simulink model "Modelo_COMPLETO_OPC"  (R2023a)
settings: Solver=ode15s  StartTime=0.0  StopTime=200  FixedStep=0.0001  MaxStep=0.01
model workspace (MAT data in the model file):
  socvcb = containers.Map
  socvcb.serialization.keys = {}
  socvcb.serialization.values = {}
  socvcb.serialization.uniformity = 0
  socvcb.serialization.keyType = 'double'
  socvcb.serialization.valueType = 'any'
undefined symbols (not defined in the file): b_cx, b_cy, b_hb, b_hd, b_hEb, b_hm, b_t, b_tb, b_td, b_tm, b_tw, b_wu, barco_x, barco_y, carro_y, constante_frenos, f, F_D_n_x, F_D_n_y, F_D_u_x, F_D_u_y, F_I_n_x, F_I_n_y, F_I_u_x, F_I_u_y, g, H_c, i_h, i_t, J_hdhEb, J_hmhb, J_td, J_tmtb, K_cy, K_tw, k_wu, M_s, M_t, muelle_x, muelle_y, pos_i_lh, pos_i_x, pos_i_yl, r_hd, r_td, riel_x, riel_y, T_hbMax, T_hEbMax, T_tbmax, xx_c0, Y_t0
libraries: simulink x6, opclib x3, vrlib x1
settings Model: Creator=Martin Tous  LastModifiedBy=Martin Tous
settings DebuggingCC: UnconnectedInputMsg=warning  UnconnectedOutputMsg=warning  UnconnectedLineMsg=warning
settings ModelReferenceCC: EnableRefExpFcnMdlSchedulingChecks=on
settings RTWCC: DLArmComputeVersion=19.05

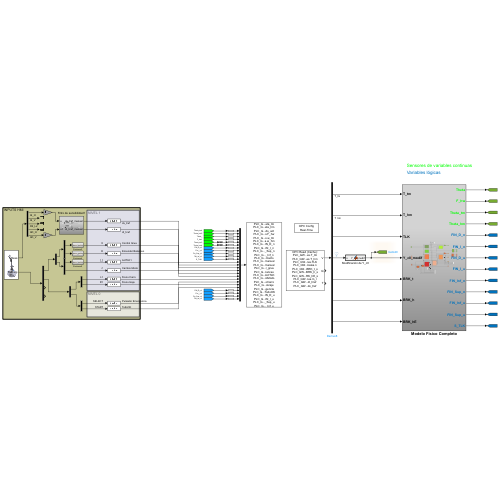
[thumbnail: Simulink's stored preview of the top-level diagram]
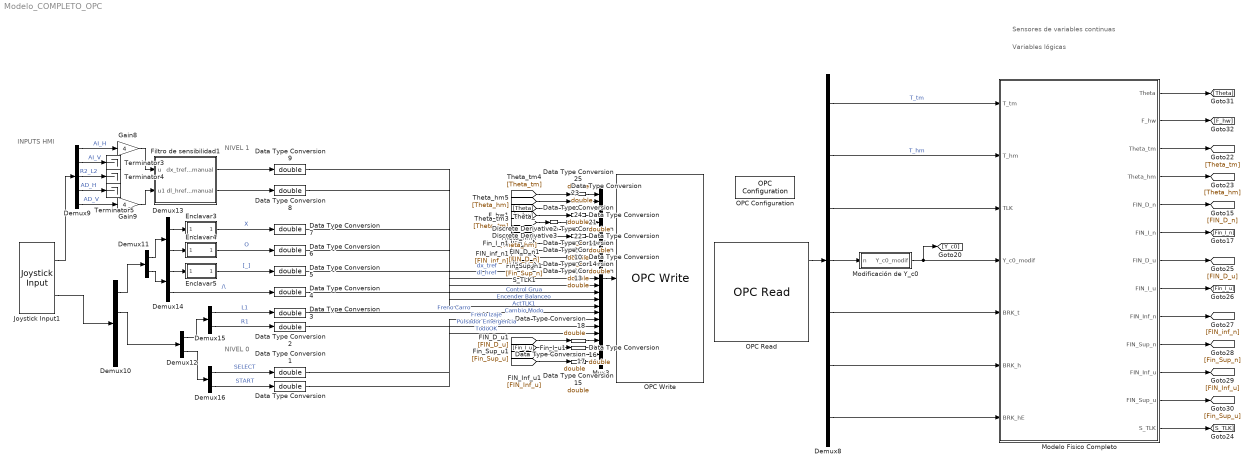
== system Modelo_COMPLETO_OPC ==
  note: INPUTS HMI
  note: NIVEL 0
  note: NIVEL 1
  note: Sensores de variables continuas
  note: Variables lógicas
  Data Type Conversion{,1..18,20..25} (25 alike) : DataTypeConversion  OutDataTypeStr=double  SaturateOnIntegerOverflow=off  RndMeth=Floor
  Demux10 : Demux
  Demux{11..16} (6 alike) : Demux  Outputs=2
  Demux8 : Demux  Outputs=7
  Demux9 : Demux  Outputs=5
  Discrete Derivative2 : simulink/Discrete/Discrete Derivative  gainval=1.0  ICPrevScaledInput=0.0  OutMin=[]  OutMax=[]  OutDataType=fixdt(1, 16)  OutScaling=2^-10  DoSatur=off
  Discrete Derivative3 : simulink/Discrete/Discrete Derivative  gainval=1.0  ICPrevScaledInput=0.0  OutMin=[]  OutMax=[]  OutDataType=fixdt(1, 16)  OutScaling=2^-10  DoSatur=off
  Enclavar3 : Stateflow chart  TreatAsAtomicUnit=on
  Enclavar4 : Stateflow chart  TreatAsAtomicUnit=on
  Enclavar5 : Stateflow chart  TreatAsAtomicUnit=on
  Filtro de sensibilidad1 : Subsystem
  Gain8 : Gain  Gain=4
  Gain9 : Gain  Gain=4
  Joystick Input1 : vrlib/Joystick Input  joyid=1  adjustports=on  forcefeed=off
  Modelo Fisico Completo : Subsystem
  Modificación de Y_c0 : MATLAB Function  TreatAsAtomicUnit=on
  Mux3 : Mux  Inputs=25
  OPC Configuration : opclib/OPC Configuration  opcServers=localhost/CoDeSys.OPC.DA/10  errMissingItems=Error  errReadWrite=Warn  errShutdown=Error  errRTViolation=Warn  rtEnable=on  speedup=1  showLatency=off  beingUsed=on
  OPC Read : opclib/OPC Read  serverHost=localhost  serverID=CoDeSys.OPC.DA  itemIDs=PLC_GW3.Application.Variables_Globales.T_tm, PLC_GW3.Application.Variables_Globales.T_hm, PLC_GW3.Application.Variables_Globales.TLK, PLC_GW3.Application.Variables_Globales.n, PLC_GW3.Application.Variables_Globales.BRK_t_s, PLC_GW3.Application.Variables_Globales.BRK_h_s, PLC_GW3.Application.Variables_Globales.BRK_hE_s, PLC_GW3.Application.Variables_Globales.m_l, PLC_GW3.Application.Variables_Globales.dl_href, PLC_GW3.Application.Variables_Globales.dx_tref  readMode=Synchronous (cache)  dataType=double  updateRate=0.01  showQual=on  showTS=on  tsMode=Seconds since start
  OPC Write : opclib/OPC Write  serverHost=localhost  serverID=CoDeSys.OPC.DA  itemIDs=PLC_GW3.Application.Variables_Globales.Theta_tm, PLC_GW3.Application.Variables_Globales.Theta_hm, PLC_GW3.Application.Variables_Globales.theta_realimentado_act, PLC_GW3.Application.Variables_Globales.F_hw, PLC_GW3.Application.Variables_Globales.w_tm, PLC_GW3.Application.Variables_Globales.w_hm, PLC_GW3.Application.Nivel1.FIN_D_n, PLC_GW3.Application.Nivel1.FIN_I_n, PLC_GW3.Application.Nivel1.FIN_Sup_n, PLC_GW3.Application.Nivel1.FIN_Inf_n, PLC_GW3.Application.Nivel1.SensoresContacto, PLC_GW3.Application.Nivel1.dx_tref_manual, PLC_GW3.Application.Nivel1.dl_href_manual, PLC_GW3.Application.Nivel1.Control_grua, PLC_GW3.Application.Nivel1.EncenderBalanceo, PLC_GW3.Application.Nivel1.ActTLK, PLC_GW3.Application.Nivel1.CambioModo, PLC_GW3.Application.Nivel1.BotonFrenoCarro, PLC_GW3.Application.Nivel1.BotonFrenoIzaje, PLC_GW3.Application.Nivel0.PulsadorEmergencia, PLC_GW3.Application.Nivel0.TodoOK, PLC_GW3.Application.Nivel0.FIN_D_u, PLC_GW3.Application.Nivel0.FIN_I_u, PLC_GW3.Application.Nivel0.FIN_Sup_u, PLC_GW3.Application.Nivel0.FIN_Inf_u  writeMode=Synchronous  updateRate=0.01
  Terminator3 : Terminator
  Terminator4 : Terminator
  Terminator5 : Terminator
  wires:
  Demux11/2 -> Demux14/1
  Demux16/1 -> Data Type Conversion1/1  "SELECT"
  Data Type Conversion3/1 -> Mux3/18  "Freno Carro"
  Data Type Conversion1/1 -> Mux3/20  "Pulsador Emergencia"
  Mux3/1 -> OPC Write/1
  Enclavar3/1(salida) -> Data Type Conversion7/1  "X"
  Filtro de sensibilidad1/1(dx_tref_manual) -> Data Type Conversion9/1
  Demux14/2 -> Data Type Conversion4/1  "/\\"
  Demux8/3 -> Modelo Fisico Completo/3(TLK)
  Demux10/1 -> Demux11/1
  Data Type Conversion6/1 -> Mux3/15  "Encender Balanceo"
  Demux14/1 -> Enclavar5/1(boton)
  Gain8/1 -> Filtro de sensibilidad1/1(u)
  Demux13/1 -> Enclavar3/1(boton)
  Demux9/3 -> Terminator4/1  "R2_L2"
  Demux9/5 -> Gain9/1  "AD_V"
  Demux13/2 -> Enclavar4/1(boton)
  Demux9/4 -> Terminator5/1  "AD_H"
  OPC Read/1 -> Demux8/1
  Gain9/1 -> Filtro de sensibilidad1/2(u1)
  Demux15/2 -> Data Type Conversion2/1  "R1"
  Demux11/1 -> Demux13/1
  Data Type Conversion7/1 -> Mux3/14  "Control Grua"
  Data Type Conversion5/1 -> Mux3/16  "ActTLK1"
  Filtro de sensibilidad1/2(dl_href_manual) -> Data Type Conversion8/1
  Demux10/2 -> Demux12/1
  Data Type Conversion2/1 -> Mux3/19  "Freno Izaje"
  Enclavar5/1(salida) -> Data Type Conversion5/1  "[_]"
  Demux12/1 -> Demux15/1
  Data Type Conversion/1 -> Mux3/21  "TodoOK"
  Demux12/2 -> Demux16/1
  Enclavar4/1(salida) -> Data Type Conversion6/1  "O"
  Demux9/2 -> Terminator3/1  "AI_V"
  Demux16/2 -> Data Type Conversion/1  "START"
  Data Type Conversion4/1 -> Mux3/17  "Cambio Modo"
  Demux9/1 -> Gain8/1  "AI_H"
  Joystick Input1/1 -> Demux9/1
  Demux15/1 -> Data Type Conversion3/1  "L1"
  Joystick Input1/2 -> Demux10/1
  [Fin_I_u] -> Data Type Conversion17/1
  [FIN_D_u] -> Data Type Conversion18/1
  [Fin_Sup_u] -> Data Type Conversion16/1
  [Fin_I_n] -> Data Type Conversion11/1
  [FIN_inf_n] -> Data Type Conversion13/1
  [Fin_Sup_n] -> Data Type Conversion12/1
  [S_TLK] -> Data Type Conversion14/1
  [FIN_D_n] -> Data Type Conversion10/1
  Data Type Conversion10/1 -> Mux3/7
  Data Type Conversion11/1 -> Mux3/8
  Data Type Conversion12/1 -> Mux3/9
  Data Type Conversion13/1 -> Mux3/10
  Data Type Conversion14/1 -> Mux3/11
  [FIN_Inf_u] -> Data Type Conversion15/1
  Data Type Conversion15/1 -> Mux3/25
  Data Type Conversion16/1 -> Mux3/24
  Data Type Conversion17/1 -> Mux3/23
  Data Type Conversion18/1 -> Mux3/22
  Discrete Derivative3/1 -> Data Type Conversion20/1
  [Theta_hm] -> Discrete Derivative3/1
  Discrete Derivative2/1 -> Data Type Conversion21/1
  [Theta_tm] -> Discrete Derivative2/1
  Data Type Conversion20/1 -> Mux3/6
  Data Type Conversion21/1 -> Mux3/5
  Data Type Conversion22/1 -> Mux3/4
  [F_hw] -> Data Type Conversion22/1
  Modelo Fisico Completo/8(FIN_I_u) -> [Fin_I_u]
  Modelo Fisico Completo/13(S_TLK) -> [S_TLK]
  Modelo Fisico Completo/5(FIN_D_n) -> [FIN_D_n]
  Modelo Fisico Completo/9(FIN_Inf_n) -> [FIN_inf_n]
  Modelo Fisico Completo/6(FIN_I_n) -> [Fin_I_n]
  Modelo Fisico Completo/2(F_hw) -> [F_hw]
  Modelo Fisico Completo/4(Theta_hm) -> [Theta_hm]
  Modelo Fisico Completo/10(FIN_Sup_n) -> [Fin_Sup_n]
  Modelo Fisico Completo/7(FIN_D_u) -> [FIN_D_u]
  Modelo Fisico Completo/1(Theta) -> [Theta]
  Modelo Fisico Completo/11(FIN_Inf_u) -> [FIN_Inf_u]
  Modelo Fisico Completo/12(FIN_Sup_u) -> [Fin_Sup_u]
  Modelo Fisico Completo/3(Theta_tm) -> [Theta_tm]
  Demux8/7 -> Modelo Fisico Completo/7(BRK_hE)
  Demux8/6 -> Modelo Fisico Completo/6(BRK_h)
  Demux8/5 -> Modelo Fisico Completo/5(BRK_t)
  Modificación de Y_c0/1(Y_c0_modif) -> Modelo Fisico Completo/4(Y_c0_modif), [Y_c0]
  [Theta] -> Data Type Conversion23/1
  Data Type Conversion23/1 -> Mux3/3
  Data Type Conversion25/1 -> Mux3/1
  Data Type Conversion24/1 -> Mux3/2
  [Theta_tm] -> Data Type Conversion25/1
  [Theta_hm] -> Data Type Conversion24/1
  Demux8/4 -> Modificación de Y_c0/1(n)
  Data Type Conversion8/1 -> Mux3/13  "dl_href"
  Data Type Conversion9/1 -> Mux3/12  "dx_tref"
  Demux8/1 -> Modelo Fisico Completo/1(T_tm)  "T_tm"
  Demux8/2 -> Modelo Fisico Completo/2(T_hm)  "T_hm"

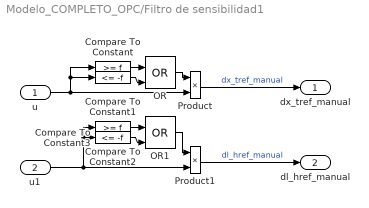
== system Modelo_COMPLETO_OPC/Filtro de sensibilidad1 ==
  u : Inport
  u1 : Inport  Port=2
  Compare To Constant : simulink/Logic and Bit Operations/Compare To Constant  relop=>=  const=f  OutDataTypeStr=boolean
  Compare To Constant1 : simulink/Logic and Bit Operations/Compare To Constant  relop=<=  const=-f  OutDataTypeStr=boolean
  Compare To Constant2 : simulink/Logic and Bit Operations/Compare To Constant  relop=>=  const=f  OutDataTypeStr=boolean
  Compare To Constant3 : simulink/Logic and Bit Operations/Compare To Constant  relop=<=  const=-f  OutDataTypeStr=boolean
  OR : Logic  Operator=OR  IconShape=distinctive  AllPortsSameDT=off  OutDataTypeStr=boolean
  OR1 : Logic  Operator=OR  IconShape=distinctive  AllPortsSameDT=off  OutDataTypeStr=boolean
  Product : Product
  Product1 : Product
  dx_tref_manual : Outport
  dl_href_manual : Outport  Port=2
  wires:
  u/1 -> Compare To Constant/1, Compare To Constant1/1, Product/2
  u1/1 -> Compare To Constant2/1, Compare To Constant3/1, Product1/2
  Compare To Constant1/1 -> OR/2
  Compare To Constant2/1 -> OR1/1
  Compare To Constant3/1 -> OR1/2
  OR1/1 -> Product1/1
  Compare To Constant/1 -> OR/1
  OR/1 -> Product/1
  Product/1 -> dx_tref_manual/1  "dx_tref_manual"
  Product1/1 -> dl_href_manual/1  "dl_href_manual"

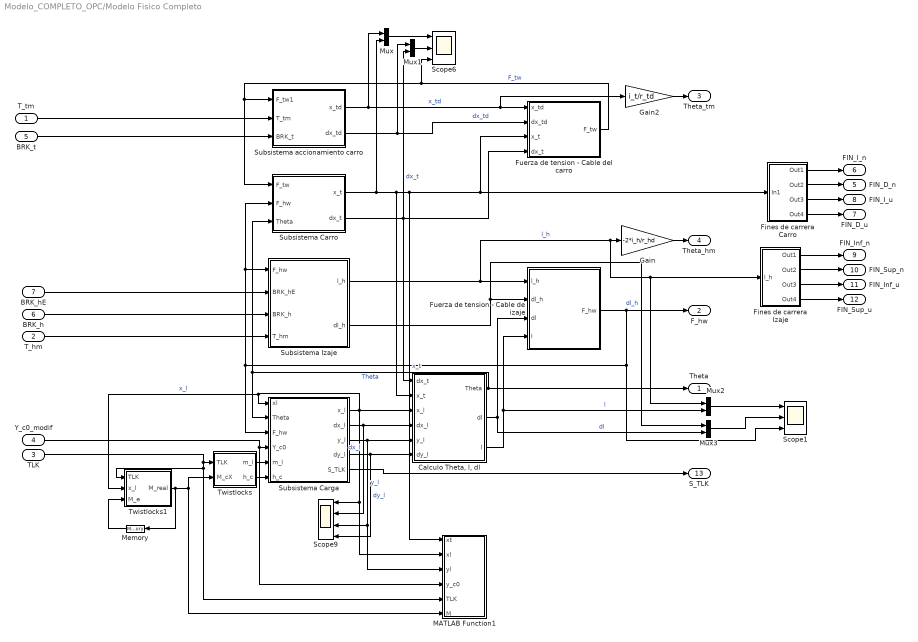
== system Modelo_COMPLETO_OPC/Modelo Fisico Completo ==
  T_tm : Inport
  T_hm : Inport  Port=2
  TLK : Inport  Port=3
  Y_c0_modif : Inport  Port=4
  BRK_t : Inport  Port=5
  BRK_h : Inport  Port=6
  BRK_hE : Inport  Port=7
  "Calculo Theta, l, dl" : Subsystem
  Fines de carrera Carro : Subsystem
  Fines de carrera Izaje : Subsystem
  Fuerza de tension - Cable de izaje : Subsystem
  Fuerza de tension - Cable del carro : Subsystem
  Gain : Gain  Gain=-2*i_h/r_hd
  Gain2 : Gain  Gain=i_t/r_td
  MATLAB Function1 : MATLAB Function  TreatAsAtomicUnit=on
  Memory : Memory
  Mux{,1..3} (4 alike) : Mux  Inputs=2
  Scope1 : Scope  NumInputPorts=3
  Scope6 : Scope  NumInputPorts=3
  Scope9 : Scope  NumInputPorts=4
  Subsistema Carga : Subsystem
  Subsistema Carro : Subsystem
  Subsistema Izaje : Subsystem
  Subsistema accionamiento carro : Subsystem
  Twistlocks : Stateflow chart  TreatAsAtomicUnit=on
  Twistlocks1 : Stateflow chart  TreatAsAtomicUnit=on
      settings: PortSchema="{\"entries\":[{\"content\":{\"sides\":[{\"content\":{\"connectorIds\":[\"In3\",\"In1\",\"In2\"]},\"type\":\"ConnectorPlacement.EquallySpacedRectSide\",\"uuid\":\"4fec8e6a-f8fa-4feb-a633-b12cd10cfa10\"},{\"content\":{\"connectorIds\":[\"Out1\"],\"side\":\"RIGHT\"},\"type\":\"ConnectorPlacement.EquallySpacedRectSide\",\"uuid\":\"3a43ccb0-d7f9-40a2-9c07-07991ad7e582\"},{\"content\":{\"connectorIds\":[],\"side\":\"TOP\"},\"type\":\"ConnectorPlacement.EquallySpacedRectSide\",\"uuid\":\"c629bb8f-87a5-4586-8b89-8bb15a2e67dc\"}]},\"type\":\"ConnectorPlacement.EquallySpacedConnector\",\"uuid\":\"e5885a79-67b0-4776-b045-dd8fc0c81e57\"}],\"packageUris\":[\"http://schema.mathworks.com/mf0/Connector/R2020b\"],\"version\":\"1.0\"}"
  Theta : Outport
  F_hw : Outport  Port=2
  Theta_tm : Outport  Port=3
  Theta_hm : Outport  Port=4
  FIN_D_n : Outport  Port=5
  FIN_I_n : Outport  Port=6
  FIN_D_u : Outport  Port=7
  FIN_I_u : Outport  Port=8
  FIN_Inf_n : Outport  Port=9
  FIN_Sup_n : Outport  Port=10
  FIN_Inf_u : Outport  Port=11
  FIN_Sup_u : Outport  Port=12
  S_TLK : Outport  Port=13
  wires:
  Fuerza de tension - Cable de izaje/1(F_hw) -> Subsistema Izaje/1(F_hw), Subsistema Carro/2(F_hw), Subsistema Carga/3(F_hw), Scope1/3, F_hw/1
  "Calculo Theta, l, dl"/1(Theta) -> Subsistema Carro/3(Theta), Subsistema Carga/2(Theta), Theta/1  "Theta"
  Subsistema Izaje/2(dl_h) -> Fuerza de tension - Cable de izaje/2(dl_h), Mux3/1  "dl_h"
  Twistlocks/1(m_l) -> Subsistema Carga/5(m_l)
  "Calculo Theta, l, dl"/2(dl) -> Mux3/2, Fuerza de tension - Cable de izaje/3(dl)  "dl"
  TLK/1 -> Twistlocks1/3(TLK), MATLAB Function1/5(TLK), Twistlocks/1(TLK)
  BRK_hE/1 -> Subsistema Izaje/2(BRK_hE)
  T_hm/1 -> Subsistema Izaje/4(T_hm)
  BRK_t/1 -> Subsistema accionamiento carro/3(BRK_t)
  BRK_h/1 -> Subsistema Izaje/3(BRK_h)
  Twistlocks/2(h_c) -> Subsistema Carga/6(h_c)
  T_tm/1 -> Subsistema accionamiento carro/2(T_tm)
  Gain2/1 -> Theta_tm/1
  Subsistema Izaje/1(l_h) -> Fuerza de tension - Cable de izaje/1(l_h), Mux2/1, Fines de carrera Izaje/1(l_h), Gain/1  "l_h"
  Gain/1 -> Theta_hm/1
  "Calculo Theta, l, dl"/3(l) -> Mux2/2, Fuerza de tension - Cable de izaje/4(l)  "l"
  Twistlocks1/1(M_real) -> Memory/1, Twistlocks/2(M_cX), MATLAB Function1/6(M)
  Subsistema Carro/2(dx_t) -> Mux1/2, Fuerza de tension - Cable del carro/4(dx_t), "Calculo Theta, l, dl"/1(dx_t)  "dx_t"
  Subsistema Carga/5(S_TLK) -> S_TLK/1
  Y_c0_modif/1 -> MATLAB Function1/4(y_c0), Subsistema Carga/4(Y_c0)
  Subsistema Carro/1(x_t) -> MATLAB Function1/1(xt), Fines de carrera Carro/1(In1), Fuerza de tension - Cable del carro/3(x_t), "Calculo Theta, l, dl"/2(x_t), Mux/2  "x_t"
  Fines de carrera Carro/1(Out1) -> FIN_I_n/1
  Fines de carrera Carro/2(Out2) -> FIN_D_n/1
  Fines de carrera Carro/3(Out3) -> FIN_I_u/1
  Fines de carrera Carro/4(Out4) -> FIN_D_u/1
  Fines de carrera Izaje/1(Out1) -> FIN_Inf_n/1
  Fines de carrera Izaje/2(Out2) -> FIN_Sup_n/1
  Fines de carrera Izaje/3(Out3) -> FIN_Inf_u/1
  Fines de carrera Izaje/4(Out4) -> FIN_Sup_u/1
  Fuerza de tension - Cable del carro/1(F_tw) -> Subsistema Carro/1(F_tw), Subsistema accionamiento carro/1(F_tw1), Scope6/3  "F_tw"
  Subsistema accionamiento carro/2(dx_td) -> Mux1/1, Fuerza de tension - Cable del carro/2(dx_td)  "dx_td"
  Subsistema accionamiento carro/1(x_td) -> Gain2/1, Fuerza de tension - Cable del carro/1(x_td), Mux/1  "x_td"
  Subsistema Carga/3(y_l) -> "Calculo Theta, l, dl"/5(y_l), Scope9/3, MATLAB Function1/3(yl)  "y_l"
  Subsistema Carga/2(dx_l) -> "Calculo Theta, l, dl"/4(dx_l), Scope9/2  "dx_l"
  Subsistema Carga/4(dy_l) -> "Calculo Theta, l, dl"/6(dy_l), Scope9/4  "dy_l"
  Subsistema Carga/1(x_l) -> "Calculo Theta, l, dl"/3(x_l), Scope9/1, MATLAB Function1/2(xl), Twistlocks1/1(x_l), Subsistema Carga/1(xl)  "x_l"
  Mux/1 -> Scope6/1
  Mux1/1 -> Scope6/2
  Mux2/1 -> Scope1/1
  Mux3/1 -> Scope1/2
  Memory/1 -> Twistlocks1/2(M_e)

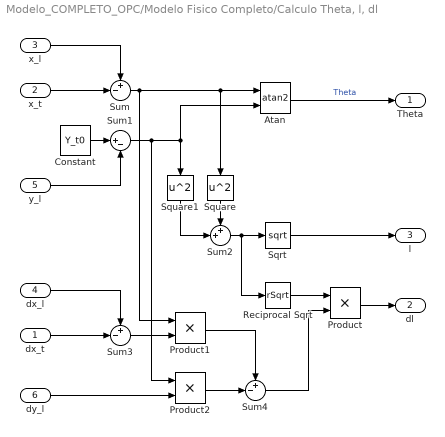
== system Modelo_COMPLETO_OPC/Modelo Fisico Completo/Calculo Theta, l, dl ==
  dx_t : Inport
  x_t : Inport  Port=2
  x_l : Inport  Port=3
  dx_l : Inport  Port=4
  y_l : Inport  Port=5
  dy_l : Inport  Port=6
  Atan : Trigonometry  Operator=atan2
  Constant : Constant  Value=Y_t0
  Product : Product
  Product1 : Product
  Product2 : Product
  Reciprocal Sqrt : Sqrt  Operator=rSqrt
  Sqrt : Sqrt
  Square : Math  Operator=square
  Square1 : Math  Operator=square
  Sum : Sum  Inputs=+-|
  Sum1 : Sum  Inputs=|+-
  Sum2 : Sum  Inputs=++|
  Sum3 : Sum  Inputs=+-|
  Sum4 : Sum  Inputs=+-|
  Theta : Outport
  dl : Outport  Port=2
  l : Outport  Port=3
  wires:
  y_l/1 -> Sum1/2
  Sum1/1 -> Product2/1, Square1/1, Atan/2
  Sum/1 -> Square/1, Atan/1, Product1/1
  Constant/1 -> Sum1/1
  Atan/1 -> Theta/1  "Theta"
  x_l/1 -> Sum/1
  x_t/1 -> Sum/2
  Square/1 -> Sum2/1
  Square1/1 -> Sum2/2
  Sum2/1 -> Reciprocal Sqrt/1, Sqrt/1
  Sqrt/1 -> l/1
  Reciprocal Sqrt/1 -> Product/1
  dx_l/1 -> Sum3/1
  dx_t/1 -> Sum3/2
  Sum3/1 -> Product1/2
  Product1/1 -> Sum4/1
  dy_l/1 -> Product2/2
  Product2/1 -> Sum4/2
  Sum4/1 -> Product/2
  Product/1 -> dl/1

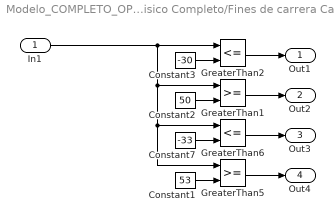
== system Modelo_COMPLETO_OPC/Modelo Fisico Completo/Fines de carrera Carro ==
  In1 : Inport
  Constant1 : Constant  Value=53
  Constant2 : Constant  Value=50
  Constant3 : Constant  Value=-30
  Constant7 : Constant  Value=-33
  GreaterThan1 : RelationalOperator  OutDataTypeStr=boolean  RndMeth=Simplest  InputSameDT=off
  GreaterThan2 : RelationalOperator  Operator=<=  OutDataTypeStr=boolean  RndMeth=Simplest  InputSameDT=off
  GreaterThan5 : RelationalOperator  OutDataTypeStr=boolean  RndMeth=Simplest  InputSameDT=off
  GreaterThan6 : RelationalOperator  Operator=<=  OutDataTypeStr=boolean  RndMeth=Simplest  InputSameDT=off
  Out1 : Outport
  Out2 : Outport  Port=2
  Out3 : Outport  Port=3
  Out4 : Outport  Port=4
  wires:
  GreaterThan1/1 -> Out2/1
  In1/1 -> GreaterThan5/1, GreaterThan6/1, GreaterThan1/1, GreaterThan2/1
  GreaterThan2/1 -> Out1/1
  Constant3/1 -> GreaterThan2/2
  Constant2/1 -> GreaterThan1/2
  Constant1/1 -> GreaterThan5/2
  Constant7/1 -> GreaterThan6/2
  GreaterThan6/1 -> Out3/1
  GreaterThan5/1 -> Out4/1

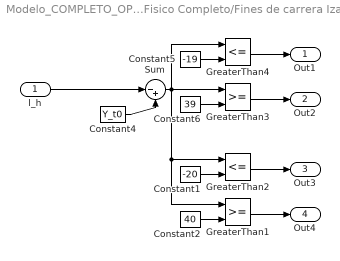
== system Modelo_COMPLETO_OPC/Modelo Fisico Completo/Fines de carrera Izaje ==
  l_h : Inport
  Constant1 : Constant  Value=-20
  Constant2 : Constant  Value=40
  Constant4 : Constant  Value=Y_t0
  Constant5 : Constant  Value=-19
  Constant6 : Constant  Value=39
  GreaterThan1 : RelationalOperator  OutDataTypeStr=boolean  RndMeth=Simplest  InputSameDT=off
  GreaterThan2 : RelationalOperator  Operator=<=  OutDataTypeStr=boolean  RndMeth=Simplest  InputSameDT=off
  GreaterThan3 : RelationalOperator  OutDataTypeStr=boolean  RndMeth=Simplest  InputSameDT=off
  GreaterThan4 : RelationalOperator  Operator=<=  OutDataTypeStr=boolean  RndMeth=Simplest  InputSameDT=off
  Sum : Sum  Inputs=|-+
  Out1 : Outport
  Out2 : Outport  Port=2
  Out3 : Outport  Port=3
  Out4 : Outport  Port=4
  wires:
  Constant1/1 -> GreaterThan2/2
  Sum/1 -> GreaterThan3/1, GreaterThan4/1, GreaterThan1/1, GreaterThan2/1
  Constant6/1 -> GreaterThan3/2
  Constant4/1 -> Sum/2
  Constant5/1 -> GreaterThan4/2
  Constant2/1 -> GreaterThan1/2
  GreaterThan3/1 -> Out2/1
  GreaterThan4/1 -> Out1/1
  l_h/1 -> Sum/1
  GreaterThan2/1 -> Out3/1
  GreaterThan1/1 -> Out4/1

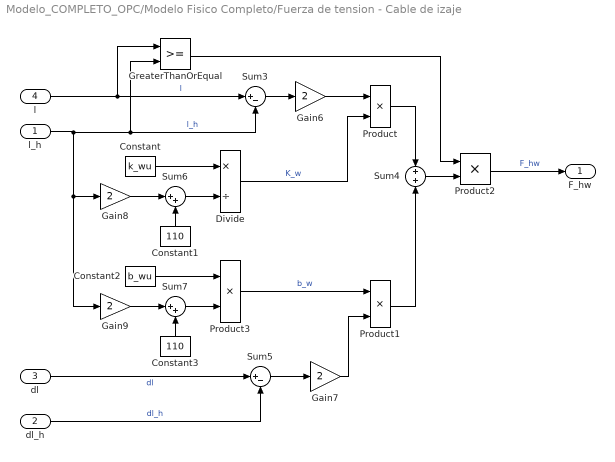
== system Modelo_COMPLETO_OPC/Modelo Fisico Completo/Fuerza de tension - Cable de izaje ==
  l_h : Inport
  dl_h : Inport  Port=2
  dl : Inport  Port=3
  l : Inport  Port=4
  Constant : Constant  Value=k_wu  SampleTime=[0, 0]
  Constant1 : Constant  Value=110
  Constant2 : Constant  Value=b_wu
  Constant3 : Constant  Value=110
  Divide : Product  Inputs=*/
  Gain{6..9} (4 alike) : Gain  Gain=2
  GreaterThanOrEqual : RelationalOperator  OutDataTypeStr=boolean  RndMeth=Simplest  InputSameDT=off
  Product{,1..3} (4 alike) : Product
  Sum3 : Sum  Inputs=|+-
  Sum4 : Sum  Inputs=+|+
  Sum5 : Sum  Inputs=|+-
  Sum6 : Sum  Inputs=|++
  Sum7 : Sum  Inputs=|++
  F_hw : Outport
  wires:
  Sum4/1 -> Product2/2
  l_h/1 -> Sum3/2, GreaterThanOrEqual/2, Gain9/1, Gain8/1  "l_h"
  Product/1 -> Sum4/1
  Sum3/1 -> Gain6/1
  Constant1/1 -> Sum6/2
  Sum6/1 -> Divide/2
  Gain6/1 -> Product/1
  l/1 -> Sum3/1, GreaterThanOrEqual/1  "l"
  Constant/1 -> Divide/1
  dl_h/1 -> Sum5/2  "dl_h"
  Sum5/1 -> Gain7/1
  Product1/1 -> Sum4/2
  GreaterThanOrEqual/1 -> Product2/1
  Product2/1 -> F_hw/1  "F_hw"
  Constant2/1 -> Product3/1
  Divide/1 -> Product/2  "K_w"
  Gain8/1 -> Sum6/1
  Constant3/1 -> Sum7/2
  Gain9/1 -> Sum7/1
  Sum7/1 -> Product3/2
  dl/1 -> Sum5/1  "dl"
  Product3/1 -> Product1/1  "b_w"
  Gain7/1 -> Product1/2

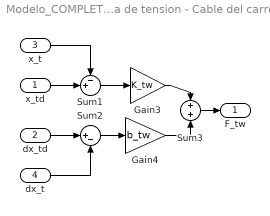
== system Modelo_COMPLETO_OPC/Modelo Fisico Completo/Fuerza de tension - Cable del carro ==
  x_td : Inport
  dx_td : Inport  Port=2
  x_t : Inport  Port=3
  dx_t : Inport  Port=4
  Gain3 : Gain  Gain=K_tw
  Gain4 : Gain  Gain=b_tw
  Sum1 : Sum  Inputs=-+|
  Sum2 : Sum  Inputs=|+-
  Sum3 : Sum  Inputs=+|+
  F_tw : Outport
  wires:
  Gain4/1 -> Sum3/2
  x_t/1 -> Sum1/1
  dx_t/1 -> Sum2/2
  dx_td/1 -> Sum2/1
  Gain3/1 -> Sum3/1
  Sum1/1 -> Gain3/1
  Sum2/1 -> Gain4/1
  x_td/1 -> Sum1/2
  Sum3/1 -> F_tw/1

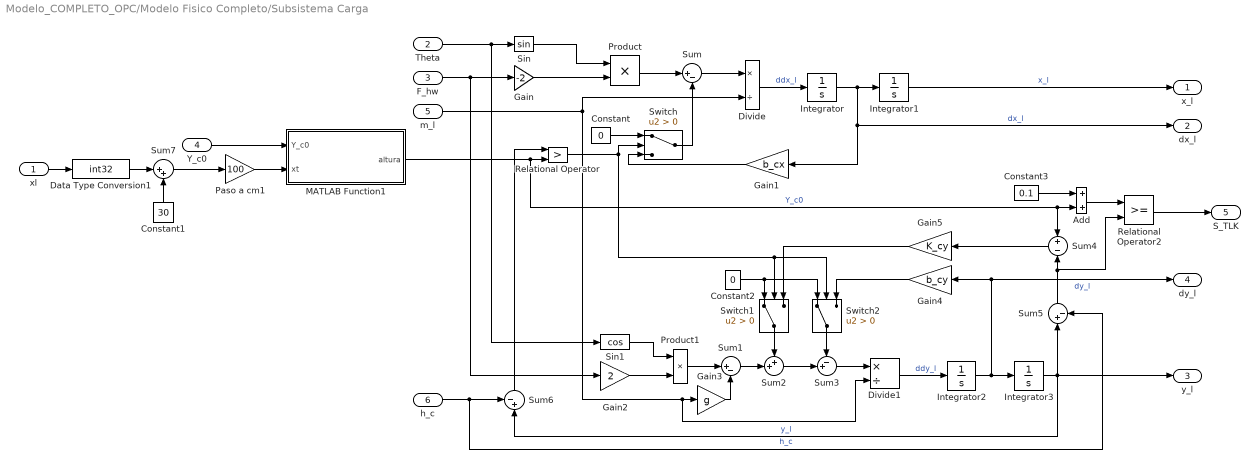
== system Modelo_COMPLETO_OPC/Modelo Fisico Completo/Subsistema Carga ==
  xl : Inport
  Theta : Inport  Port=2
  F_hw : Inport  Port=3
  Y_c0 : Inport  Port=4
  m_l : Inport  Port=5
  h_c : Inport  Port=6
  Add : Sum
  Constant : Constant  Value=0
  Constant1 : Constant  Value=30
  Constant2 : Constant  Value=0
  Constant3 : Constant  Value=0.1
  Data Type Conversion1 : DataTypeConversion  OutDataTypeStr=int32  SaturateOnIntegerOverflow=off  RndMeth=Floor
  Divide : Product  Inputs=*/
  Divide1 : Product  Inputs=*/
  Gain : Gain  Gain=-2
  Gain1 : Gain  Gain=b_cx
  Gain2 : Gain  Gain=2
  Gain3 : Gain  Gain=g
  Gain4 : Gain  Gain=b_cy
  Gain5 : Gain  Gain=K_cy
  Integrator : Integrator
  Integrator1 : Integrator  InitialCondition=pos_i_x
  Integrator2 : Integrator
  Integrator3 : Integrator  InitialCondition=pos_i_yl
  MATLAB Function1 : MATLAB Function  TreatAsAtomicUnit=on
  Paso a cm1 : Gain  Gain=100
  Product : Product
  Product1 : Product
  Relational Operator : RelationalOperator  Operator=>  OutDataTypeStr=boolean  RndMeth=Simplest  InputSameDT=off
  Relational Operator2 : RelationalOperator  OutDataTypeStr=boolean  RndMeth=Simplest  InputSameDT=off
  Sin : Trigonometry
  Sin1 : Trigonometry  Operator=cos
  Sum : Sum  Inputs=|+-
  Sum1 : Sum  Inputs=|+-
  Sum2 : Sum  Inputs=++|
  Sum3 : Sum  Inputs=-+|
  Sum4 : Sum  Inputs=+|-
  Sum5 : Sum  Inputs=|+-
  Sum6 : Sum  Inputs=-+|
  Sum7 : Sum  Inputs=|++
  Switch : Switch  Criteria=u2 > Threshold  SaturateOnIntegerOverflow=off  InputSameDT=off
  Switch1 : Switch  Criteria=u2 > Threshold  SaturateOnIntegerOverflow=off  InputSameDT=off
  Switch2 : Switch  Criteria=u2 > Threshold  SaturateOnIntegerOverflow=off  InputSameDT=off
  x_l : Outport
  dx_l : Outport  Port=2
  y_l : Outport  Port=3
  dy_l : Outport  Port=4
  S_TLK : Outport  Port=5
  wires:
  Integrator3/1 -> y_l/1, Sum6/2, Sum5/1  "y_l"
  Relational Operator/1 -> Switch2/2, Switch1/2, Switch/2
  Divide/1 -> Integrator/1  "ddx_l"
  Switch2/1 -> Sum3/1
  Integrator/1 -> dx_l/1, Gain1/1, Integrator1/1  "dx_l"
  h_c/1 -> Sum5/2, Sum6/1  "h_c"
  Gain3/1 -> Sum1/2
  F_hw/1 -> Gain/1, Gain2/1
  Product/1 -> Sum/1
  Switch1/1 -> Sum2/1
  Sum6/1 -> Relational Operator/1
  Sum1/1 -> Sum2/2
  Gain1/1 -> Switch/3
  Integrator2/1 -> dy_l/1, Gain4/1, Integrator3/1  "dy_l"
  Gain/1 -> Product/2
  Gain5/1 -> Switch1/3
  Sin1/1 -> Product1/1
  Sin/1 -> Product/1
  Sum/1 -> Divide/1
  Integrator1/1 -> x_l/1  "x_l"
  Gain4/1 -> Switch2/3
  Sum5/1 -> Relational Operator2/2, Sum4/2
  Sum4/1 -> Gain5/1
  Theta/1 -> Sin/1, Sin1/1
  Constant2/1 -> Switch2/1, Switch1/1
  Divide1/1 -> Integrator2/1  "ddy_l"
  Gain2/1 -> Product1/2
  Product1/1 -> Sum1/1
  m_l/1 -> Divide/2, Divide1/2, Gain3/1
  Sum2/1 -> Sum3/2
  Sum3/1 -> Divide1/1
  Constant/1 -> Switch/1
  Switch/1 -> Sum/2
  MATLAB Function1/1(altura) -> Sum4/1, Add/2, Relational Operator/2  "Y_c0"
  Relational Operator2/1 -> S_TLK/1
  Paso a cm1/1 -> MATLAB Function1/2(xt)
  Y_c0/1 -> MATLAB Function1/1(Y_c0)
  xl/1 -> Data Type Conversion1/1
  Sum7/1 -> Paso a cm1/1
  Constant1/1 -> Sum7/2
  Data Type Conversion1/1 -> Sum7/1
  Add/1 -> Relational Operator2/1
  Constant3/1 -> Add/1

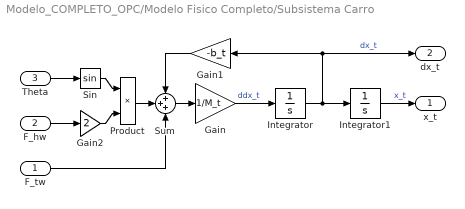
== system Modelo_COMPLETO_OPC/Modelo Fisico Completo/Subsistema Carro ==
  F_tw : Inport
  F_hw : Inport  Port=2
  Theta : Inport  Port=3
  Gain : Gain  Gain=1/M_t
  Gain1 : Gain  Gain=-b_t
  Gain2 : Gain  Gain=2
  Integrator : Integrator
  Integrator1 : Integrator  InitialCondition=pos_i_x
  Product : Product
  Sin : Trigonometry
  Sum : Sum  Inputs=+++
  x_t : Outport
  dx_t : Outport  Port=2
  wires:
  Sin/1 -> Product/1
  Gain2/1 -> Product/2
  F_hw/1 -> Gain2/1
  Integrator/1 -> Integrator1/1, dx_t/1, Gain1/1  "dx_t"
  Gain1/1 -> Sum/1
  Integrator1/1 -> x_t/1  "x_t"
  Product/1 -> Sum/2
  Gain/1 -> Integrator/1  "ddx_t"
  Sum/1 -> Gain/1
  Theta/1 -> Sin/1
  F_tw/1 -> Sum/3

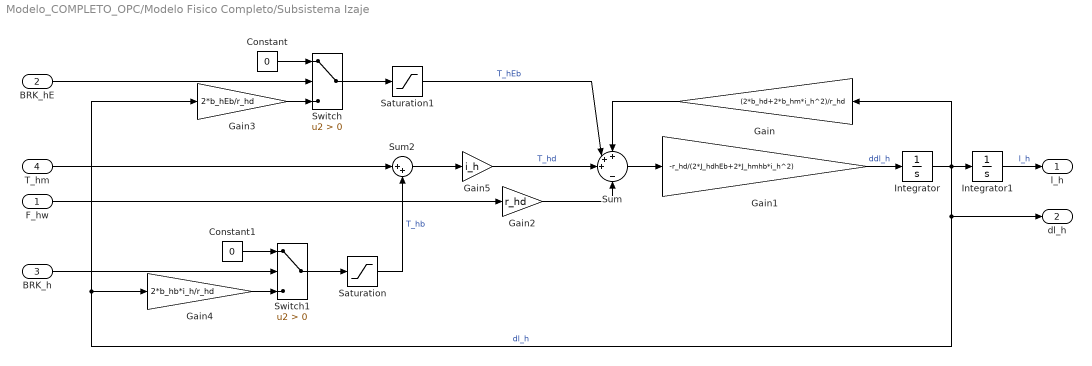
== system Modelo_COMPLETO_OPC/Modelo Fisico Completo/Subsistema Izaje ==
  F_hw : Inport
  BRK_hE : Inport  Port=2
  BRK_h : Inport  Port=3
  T_hm : Inport  Port=4
  Constant : Constant  Value=0
  Constant1 : Constant  Value=0
  Gain : Gain  Gain=(2*b_hd+2*b_hm*i_h^2)/r_hd
  Gain1 : Gain  Gain=-r_hd/(2*J_hdhEb+2*J_hmhb*i_h^2)
  Gain2 : Gain  Gain=r_hd
  Gain3 : Gain  Gain=2*b_hEb/r_hd
  Gain4 : Gain  Gain=2*b_hb*i_h/r_hd
  Gain5 : Gain  Gain=i_h
  Integrator : Integrator
  Integrator1 : Integrator  InitialCondition=pos_i_lh
  Saturation : Saturate  UpperLimit=T_hbMax*constante_frenos  LowerLimit=-T_hbMax*constante_frenos
  Saturation1 : Saturate  UpperLimit=T_hEbMax*constante_frenos  LowerLimit=-T_hEbMax*constante_frenos
  Sum : Sum  Inputs=+++|-
  Sum2 : Sum  Inputs=|++
  Switch : Switch  Criteria=u2 > Threshold  SaturateOnIntegerOverflow=off  InputSameDT=off
  Switch1 : Switch  Criteria=u2 > Threshold  SaturateOnIntegerOverflow=off  InputSameDT=off
  l_h : Outport
  dl_h : Outport  Port=2
  wires:
  T_hm/1 -> Sum2/1
  Saturation1/1 -> Sum/2  "T_hEb"
  Gain/1 -> Sum/1
  Gain1/1 -> Integrator/1  "ddl_h"
  Sum/1 -> Gain1/1
  Gain5/1 -> Sum/3  "T_hd"
  Integrator1/1 -> l_h/1  "l_h"
  Sum2/1 -> Gain5/1
  F_hw/1 -> Gain2/1
  Switch/1 -> Saturation1/1
  Saturation/1 -> Sum2/2  "T_hb"
  Gain2/1 -> Sum/4
  Integrator/1 -> dl_h/1, Gain3/1, Gain4/1, Gain/1, Integrator1/1  "dl_h"
  BRK_hE/1 -> Switch/2
  Gain3/1 -> Switch/3
  Constant/1 -> Switch/1
  Constant1/1 -> Switch1/1
  BRK_h/1 -> Switch1/2
  Gain4/1 -> Switch1/3
  Switch1/1 -> Saturation/1

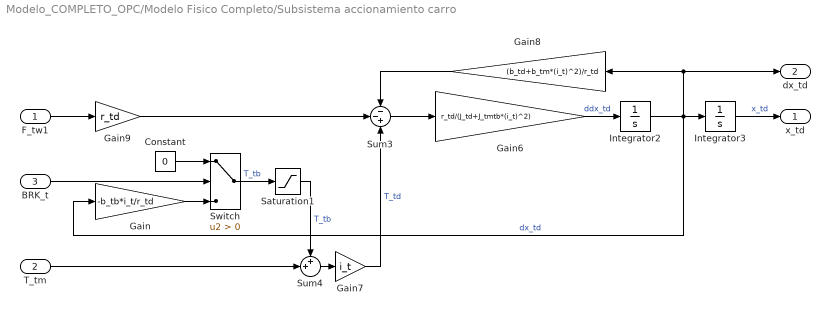
== system Modelo_COMPLETO_OPC/Modelo Fisico Completo/Subsistema accionamiento carro ==
  F_tw1 : Inport
  T_tm : Inport  Port=2
  BRK_t : Inport  Port=3
  Constant : Constant  Value=0
  Gain : Gain  Gain=-b_tb*i_t/r_td
  Gain6 : Gain  Gain=r_td/(J_td+J_tmtb*(i_t)^2)
  Gain7 : Gain  Gain=i_t
  Gain8 : Gain  Gain=(b_td+b_tm*(i_t)^2)/r_td
  Gain9 : Gain  Gain=r_td
  Integrator2 : Integrator
  Integrator3 : Integrator  InitialCondition=pos_i_x
  Saturation1 : Saturate  UpperLimit=T_tbmax*constante_frenos  LowerLimit=-T_tbmax*constante_frenos
  Sum3 : Sum  Inputs=--+
  Sum4 : Sum  Inputs=++|
  Switch : Switch  Criteria=u2 > Threshold  SaturateOnIntegerOverflow=off  InputSameDT=off
  x_td : Outport
  dx_td : Outport  Port=2
  wires:
  Switch/1 -> Saturation1/1  "T_tb"
  F_tw1/1 -> Gain9/1
  Sum3/1 -> Gain6/1
  Gain7/1 -> Sum3/3  "T_td"
  Gain8/1 -> Sum3/1
  Integrator2/1 -> Gain8/1, dx_td/1, Gain/1, Integrator3/1  "dx_td"
  Sum4/1 -> Gain7/1
  Gain6/1 -> Integrator2/1  "ddx_td"
  Gain9/1 -> Sum3/2
  T_tm/1 -> Sum4/2
  Integrator3/1 -> x_td/1  "x_td"
  Constant/1 -> Switch/1
  Gain/1 -> Switch/3
  BRK_t/1 -> Switch/2
  Saturation1/1 -> Sum4/1  "T_tb"

== matlab function Modelo_COMPLETO_OPC/Modelo Fisico Completo/Subsistema Carga/MATLAB Function1 ==
  data: Y_c0 input; xt input; altura output
function altura = Perfil_de_Obstaculos(Y_c0, xt)

% Ingreso el valor de x (en cm) para el que quiero saber Y_c0
if xt<=100 || xt>=8000
    altura=0;
else
    altura = Y_c0(xt);
end 

end

== stateflow chart Modelo_COMPLETO_OPC/Modelo Fisico Completo/Twistlocks ==
  (default) -> (junction 7) : % Modos de Twistlocks
  (junction 7) -> (junction 8) [order 1] : [TLK == 0]
  (junction 7) -> (junction 9) [order 2] : {h_c = H_c; m_l = M_s+M_cX;}
  (junction 8) -> (junction 10) : {h_c = 0; m_l = M_s;}
  (junction 10) -> (junction 9)
  (junction 9) -> (junction 11)
  data: H_c parameter; M_s parameter; TLK input; m_l output; h_c output; M_cX input

== stateflow chart Modelo_COMPLETO_OPC/Modelo Fisico Completo/Twistlocks1 ==
  (default) -> (junction 20) : % Modos de Twistlocks
  (junction 20) -> (junction 22) [order 2] : [TLK==1]
  (junction 22) -> (junction 24) : {M_real=M_e;}
  (junction 20) -> (junction 7) [order 1] : [TLK==0]
  (junction 7) -> (junction 8) [order 1] : [x_l <= -7.5 && x_l>=-10]
  (junction 7) -> (junction 9) [order 2] : {M_real=40000;}
  (junction 8) -> (junction 10) : {M_real=80000;}
  (junction 24) -> (junction 9)
  (junction 10) -> (junction 9)
  (junction 9) -> (junction 11)
  data: x_l input; M_real output; M_e input; TLK input

== matlab function Modelo_COMPLETO_OPC/Modificación de Y_c0 ==
  data: n input; Y_c0_modif output; Y_c0 parameter

function Y_c0_modif = fcn(n, Y_c0)

persistent y
persistent n_ant
if isempty(y)
    n_ant=0;
    Y_c0_modif = Y_c0;
    if n~=500 && n~= n_ant
        Y_c0_modif(250*abs(n)-249:250*abs(n)) = Y_c0(250*abs(n)-249:250*abs(n))+sign(n)*2.5;
    end
        y=Y_c0_modif;
else
    Y_c0_modif = y;
    if n~=500 && n ~= n_ant
        Y_c0_modif(250*abs(n)-249:250*abs(n)) = y(250*abs(n)-249:250*abs(n))+sign(n)*2.5;
    end
        y=Y_c0_modif;
end
n_ant=n;

== stateflow chart Modelo_COMPLETO_OPC/Enclavar3 ==
  state Espera
  state Cambiar
    entry:
    salida=(~salida);
  (default) -> Espera
  Espera -> Cambiar : [boton]
  Cambiar -> Espera : [boton==0]
  data: boton input; salida output boolean =false

== stateflow chart Modelo_COMPLETO_OPC/Enclavar4 ==
  state Espera
  state Cambiar
    entry:
    salida=(~salida);
  (default) -> Espera
  Espera -> Cambiar : [boton]
  Cambiar -> Espera : [boton==0]
  data: boton input; salida output boolean =false

== stateflow chart Modelo_COMPLETO_OPC/Enclavar5 ==
  state Espera
  state Cambiar
    entry:
    salida=(~salida);
  (default) -> Espera
  Espera -> Cambiar : [boton]
  Cambiar -> Espera : [boton==0]
  data: boton input; salida output boolean =false

== matlab function Modelo_COMPLETO_OPC/Modelo Fisico Completo/MATLAB Function1 ==
  settings: updateMethod=DISCRETE
  data: xt input; xl input; yl input; y_c0 input; TLK input; M input; barco_y parameter; barco_x parameter; muelle_y parameter; muelle_x parameter; riel_y parameter; riel_x parameter; carro_y parameter; xx_c0 parameter; F_I_n_x parameter; F_I_n_y parameter; F_I_u_x parameter; F_I_u_y parameter; F_D_n_x parameter; F_D_n_y parameter; F_D_u_x parameter; F_D_u_y parameter
function fcn(xt,xl, yl, y_c0,TLK, M, barco_y, barco_x, muelle_y, muelle_x, riel_y, riel_x, carro_y, xx_c0, F_I_n_x, F_I_n_y, F_I_u_x, F_I_u_y, F_D_n_x, F_D_n_y, F_D_u_x, F_D_u_y)
    persistent fig
    persistent trayectoria
    persistent spreader
    persistent y_c0_previo
    persistent carro
    persistent cable
    persistent perfil
    persistent contenedor
    persistent contenedor_pesado
    persistent y_ant
    
    carro_x = (xt-1):0.1:(xt+0.9);
    
    spreader_x = (xl-1.25):0.1:(xl+1.15);
    spreader_y = ones(1, length(spreader_x)) * yl;
    
    contenedor_x = (xl-1.25):0.1:(xl+1.15);
    contenedor_y = ones(1, length(contenedor_x)) * (yl-1.25);
    
    contenedor_pesado_x = -10:0.1:-7.5;
    contenedor_pesado_y= ones(1,length(contenedor_pesado_x))*1.25;
    
    cable_y=45:-0.1:yl;
    long_cable=length(cable_y);
    cable_x=ones(1,length(cable_y));
    
    if xl==xt
        cable_x=cable_x*xt;
    elseif xt>xl
        dx_l=(xt-xl)/long_cable;
        cable_x=xt:-dx_l:(xl+dx_l);
    else 
        dx_l=(xl-xt)/long_cable;
        cable_x=xt:dx_l:(xl-dx_l);
    end 
    
    if isempty(fig)
        fig = figure(8);
        trayectoria = plot(xl, yl, 'LineWidth', 1.5);
        xlim([-35 55])
        ylim([-20 50])
        grid on
        grid minor
        hold on
        y_ant=y_c0;
        y_c0_previo = plot(xx_c0, y_c0, 'c', 'LineWidth', 2);
        perfil=plot(xx_c0, y_c0, 'r', 'LineWidth', 2);
        plot(riel_x, riel_y, 'bx', 'LineWidth', 1)
        carro = plot(carro_x, carro_y,'k', 'LineWidth', 10);
        cable = plot(cable_x, cable_y,'k');
        spreader = plot(spreader_x, spreader_y, 'k', 'LineWidth', 2);
        contenedor = plot(-50, 0, 'y', 'LineWidth', 10);
        contenedor_pesado = plot(contenedor_pesado_x, contenedor_pesado_y, 'r', 'LineWidth', 10);
        plot(muelle_x, muelle_y, 'k', 'LineWidth', 2)
        plot(barco_x, barco_y, 'b', 'LineWidth', 2)
        plot(F_I_n_x, F_I_n_y, 'r', 'LineWidth', 1.5)
        plot(F_I_u_x, F_I_u_y, 'r', 'LineWidth', 1.5)
        plot(F_D_n_x, F_D_n_y, 'r', 'LineWidth', 1.5)
        plot(F_D_u_x, F_D_u_y, 'r', 'LineWidth', 1.5)
        
        hold off
    else
        set(trayectoria, 'XData', [get(trayectoria, 'XData'), xl], 'YData', [get(trayectoria, 'YData'), yl])
        set(spreader, 'XData', spreader_x, 'YData', spreader_y)
        set(carro, 'XData', carro_x, 'YData', carro_y)
        set(cable, 'XData', cable_x, 'YData', cable_y)
            
        if TLK==1
            if M==80000
                set(contenedor_pesado, 'XData', contenedor_x, 'YData', contenedor_y)
            else
            set(contenedor, 'XData', contenedor_x, 'YData', contenedor_y)
            end
        end
        if ~isequal(y_ant, y_c0)  
            set(perfil,'YData', y_c0)
            set(y_c0_previo,'YData', y_ant)
            y_ant = y_c0;
        end
        
    end
end
